simulink model "lqr_1dof_nonlinear_speed"  (R2017a)
settings: Solver=ode45  StartTime=0.0  StopTime=10  RelTol=1e-3
undefined symbols (not defined in the file): f, g, J, K, k_p, L, l, m_p
settings Model: Creator=sansh  LastModifiedBy=rj2318

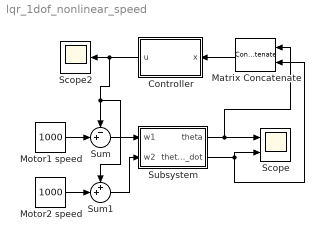
== system lqr_1dof_nonlinear_speed ==
  Controller : Subsystem
  Matrix Concatenate : Concatenate  Mode=Multidimensional array  ConcatenateDimension=2
  Motor1 speed : Constant  Value=1000
  Motor2 speed : Constant  Value=1000
  Scope : Scope  NumInputPorts=2
  Scope2 : Scope
  Subsystem : Subsystem
  Sum : Sum  Inputs=-+|
  Sum1 : Sum  Inputs=++|
  wires:
  Subsystem/1(theta) -> Matrix Concatenate/1, Scope/1
  Subsystem/2(theta_dot) -> Scope/2, Matrix Concatenate/2
  Matrix Concatenate/1 -> Controller/1(x)
  Sum1/1 -> Subsystem/2(w2)
  Motor2 speed/1 -> Sum1/2
  Controller/1(u) -> Sum1/1, Sum/1, Scope2/1
  Motor1 speed/1 -> Sum/2
  Sum/1 -> Subsystem/1(w1)

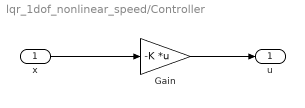
== system lqr_1dof_nonlinear_speed/Controller ==
  x : Inport
  Gain : Gain  Gain=-K  Multiplication=Matrix(K*u)
  u : Outport
  wires:
  Gain/1 -> u/1
  x/1 -> Gain/1

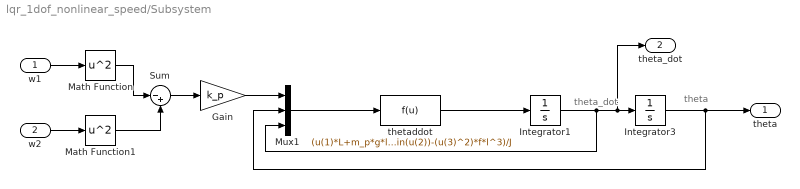
== system lqr_1dof_nonlinear_speed/Subsystem ==
  note: theta
  note: theta_dot
  w1 : Inport
  w2 : Inport  Port=2
  Gain : Gain  Gain=k_p
  Integrator1 : Integrator  ContinuousStateAttributes='thetadot'
  Integrator3 : Integrator  InitialCondition=0.1  ContinuousStateAttributes='theta'
  Math Function : Math  Operator=square  SaturateOnIntegerOverflow=on
  Math Function1 : Math  Operator=square  SaturateOnIntegerOverflow=on
  Mux1 : Mux  Inputs=3
  Sum : Sum  Inputs=|-+
  thetaddot : Fcn  Expr=(u(1)*L+m_p*g*l*sin(u(2))-(u(3)^2)*f*l^3)/J
  theta : Outport
  theta_dot : Outport  Port=2
  wires:
  Mux1/1 -> thetaddot/1
  thetaddot/1 -> Integrator1/1
  Integrator1/1 -> Mux1/3, theta_dot/1, Integrator3/1
  Integrator3/1 -> Mux1/2, theta/1
  Math Function/1 -> Sum/1
  w1/1 -> Math Function/1
  Math Function1/1 -> Sum/2
  Sum/1 -> Gain/1
  w2/1 -> Math Function1/1
  Gain/1 -> Mux1/1
